simulink model "IntegA"  (Simulink 7.2)
settings: Solver=ode45  StartTime=0.0  StopTime=10.0  RelTol=1e-3
settings Model: Creator=FVOliveira  LastModifiedBy=FVOliveira

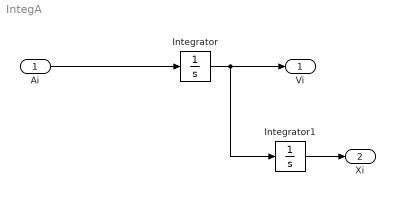
== system IntegA ==
  Ai : Inport  OutDataType=sfix(16)  OutScaling=2^0
  Integrator : Integrator
  Integrator1 : Integrator
  Vi : Outport  OutDataType=sfix(16)  OutScaling=2^0
  Xi : Outport  Port=2  OutDataType=sfix(16)  OutScaling=2^0
  wires:
  Ai/1 -> Integrator/1
  Integrator/1 -> Vi/1, Integrator1/1
  Integrator1/1 -> Xi/1
